simulink model "celp_ex_lsf"  (Simulink 6.1)
settings: Solver=FixedStepDiscrete  SolverMode=SingleTasking  StartTime=0.0  StopTime=300  RelTol=1e-3
PreLoadFcn:
  | load lpcvocoder.mat;
undefined symbols (not defined in the file): jet, magnitude, poly2lsf
libraries: simulink x16, dspcelplib x12, dspindex x9, dspstat3 x8, dspbuff3 x8, dspquant2 x6, dspmtrx3 x6, dsparch4 x4, dspsigops x4, dspmathops x4, dsplp x3, dspspect3 x3
(part 2 of 2)

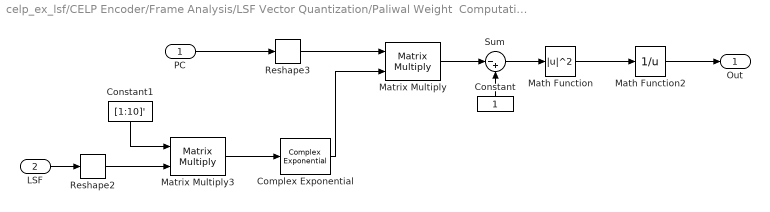
== system celp_ex_lsf/CELP Encoder/Frame Analysis/LSF Vector Quantization/Paliwal Weight  Computation/LPCpowSpec ==
  PC : Inport  Port=1  LatchInput=off
  LSF : Inport  Port=2  LatchInput=off
  Complex Exponential : dspmathops/Complex Exponential
  Constant : Constant  Orientation=up  VectorParams1D=off  SampleTime=-1
  Constant1 : Constant  Orientation=down  Value=[1:10]'  VectorParams1D=off  SampleTime=-1
  Math Function : Math  Operator=magnitude^2  SaturateOnIntegerOverflow=on
  Math Function2 : Math  Operator=reciprocal  SaturateOnIntegerOverflow=on
  Matrix Multiply : dspmtrx3/Matrix Multiply  numInputPorts=2  OptimizationLevel=None
  Matrix Multiply3 : dspmtrx3/Matrix Multiply  numInputPorts=2  OptimizationLevel=None
  Reshape2 : simulink/Math Operations/Reshape  OutputDimensionality=Row vector  OutputDimensions=[1,1]
  Reshape3 : simulink/Math Operations/Reshape  OutputDimensionality=Row vector  OutputDimensions=[1,1]
  Sum : Sum  Inputs=|-+  SaturateOnIntegerOverflow=on
  Out : Outport
  wires:
  Math Function2/1 -> Out/1
  Matrix Multiply/1 -> Sum/1
  PC/1 -> Reshape3/1
  Complex Exponential/1 -> Matrix Multiply/2
  Math Function/1 -> Math Function2/1
  Sum/1 -> Math Function/1
  Constant/1 -> Sum/2
  Reshape3/1 -> Matrix Multiply/1
  LSF/1 -> Reshape2/1
  Reshape2/1 -> Matrix Multiply3/2
  Constant1/1 -> Matrix Multiply3/1
  Matrix Multiply3/1 -> Complex Exponential/1

== system celp_ex_lsf/CELP Encoder/Subframe Analysis/Innovation signal quantization/Impulse Response/For Iterator Subsystem2 ==
  SigIn2 : Inport  Port=1  LatchInput=off
  K : Inport  Port=2  LatchInput=off
  For Iterator : ForIterator  ResetStates=reset  IterationLimit=1  ShowIterationPort=off
  Time-Varying  Synthesis Filter 1/A(z). : dsparch4/Digital Filter  DialogController=dspDDGCreate  DialogControllerArgs=DataTag6  TypePopup=IIR (all poles)  IIRFiltStruct=Direct form II transposed  AllPoleFiltStruct=Lattice AR  FIRFiltStruct=Direct form  CoeffSource=Input port(s)  NumCoeffs=[1 -.95]  DenCoeffs=[1 0.1]  BiQuadCoeffs=[1 0.3 0.4 1 0.1 0.2]  LatticeCoeffs=[0.2 0.4]  denIgnore=off  FiltPerSampPopup=One filter per frame  IC=0  ICnum=0  ICden=0  roundingMode=Floor  overflowMode=off  ScaleValues=1  scaleValueFracLength=14  stageInFracLength=15  stageOutFracLength=15
  SigOut2 : Outport
  wires:
  K/1 -> Time-Varying  Synthesis Filter 1/A(z)./2
  SigIn2/1 -> Time-Varying  Synthesis Filter 1/A(z)./1
  Time-Varying  Synthesis Filter 1/A(z)./1 -> SigOut2/1

== system celp_ex_lsf/CELP Encoder/Subframe Analysis/Innovation signal quantization/Searching for FCB pulse  positions and FCB gain/  ==
  note: This subsystem finds four FCB pulse positions and the
      | sign of the corresponding pulses based on the error between
      | the original pitch residual and its quantized version.

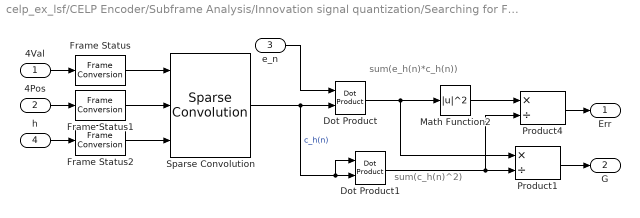
== system celp_ex_lsf/CELP Encoder/Subframe Analysis/Innovation signal quantization/Searching for FCB pulse  positions and FCB gain/Computation of  Error and Gain ==
  note: sum(e_h(n)*c_h(n))
  note: sum(c_h(n)^2)
  4Val : Inport  Port=1  LatchInput=off
  4Pos : Inport  Port=2  LatchInput=off
  e_n : Inport  Port=3  LatchInput=off
  h : Inport  Port=4  LatchInput=off
  Dot Product : simulink/Math Operations/Dot Product  OutDataType=sfix(16)  OutScaling=2^-10  DoSatur=on
  Dot Product1 : simulink/Math Operations/Dot Product  OutDataType=sfix(16)  OutScaling=2^-10  DoSatur=on
  Frame Status : FrameConversion
  Frame Status1 : FrameConversion
  Frame Status2 : FrameConversion
  Math Function2 : Math  Operator=magnitude^2  SaturateOnIntegerOverflow=on
  Product1 : Product  Inputs=*/  SaturateOnIntegerOverflow=on
  Product4 : Product  Inputs=*/  SaturateOnIntegerOverflow=on
  Sparse Convolution : dspcelplib/Sparse Convolution
  Err : Outport
  G : Outport  Port=2
  wires:
  Dot Product1/1 -> Product4/2, Product1/2
  Math Function2/1 -> Product4/1
  Dot Product/1 -> Math Function2/1, Product1/1
  Sparse Convolution/1 -> Dot Product/2, Dot Product1/2, Dot Product1/1  "c_h(n)"
  e_n/1 -> Dot Product/1
  4Val/1 -> Frame Status/1
  Product4/1 -> Err/1
  4Pos/1 -> Frame Status1/1
  h/1 -> Frame Status2/1
  Product1/1 -> G/1
  Frame Status/1 -> Sparse Convolution/1
  Frame Status1/1 -> Sparse Convolution/2
  Frame Status2/1 -> Sparse Convolution/3

== system celp_ex_lsf/CELP Encoder/Subframe Analysis/Innovation signal quantization/Searching for FCB pulse  positions and FCB gain/Optimal Features ==
  SignBit : Inport  Port=1  LatchInput=off
  Err : Inport  Port=2  LatchInput=off
  G : Inport  Port=3  LatchInput=off
  Pos : Inport  Port=4  LatchInput=off
  Data Type Conversion : DataTypeConversion  OutDataTypeMode=double  SaturateOnIntegerOverflow=on  RndMeth=Zero
  Data Type Conversion1 : DataTypeConversion  OutDataTypeMode=double  SaturateOnIntegerOverflow=on  RndMeth=Zero
  Delay1 : dspsigops/Delay  Orientation=left  dly_unit=Frames  delay=1  ic_detail=on  dif_ic_for_ch=off  dif_ic_for_dly=off  ic=0  reset_popup=None
  Feature  Concatenation : simulink/Math Operations/Matrix Concatenation  numInports=3  catMethod=Vertical
  Local maxima detector : Subsystem
  Switch : Switch  Criteria=u2 ~= 0  InputSameDT=on
  Features : Outport
  wires:
  Local maxima detector/1(Flag) -> Switch/2
  Switch/1 -> Delay1/1, Features/1
  Delay1/1 -> Switch/3
  Feature  Concatenation/1 -> Switch/1
  Data Type Conversion/1 -> Feature  Concatenation/1
  Data Type Conversion1/1 -> Feature  Concatenation/2
  Pos/1 -> Data Type Conversion/1
  SignBit/1 -> Data Type Conversion1/1
  G/1 -> Feature  Concatenation/3
  Err/1 -> Local maxima detector/1(Err)

== system celp_ex_lsf/CELP Encoder/Subframe Analysis/Innovation signal quantization/Searching for FCB pulse  positions and FCB gain/Partial decomposition of  Pitch Residual ==
  PitchRes : Inport  Port=1  LatchInput=off
  Idx : Inport  Port=2  LatchInput=off
  Control : Inport  Port=3  LatchInput=off
  Data Type Conversion : DataTypeConversion  OutDataTypeMode=double  SaturateOnIntegerOverflow=on  RndMeth=Zero
  Data Type Conversion1 : DataTypeConversion  OutDataTypeMode=int32  SaturateOnIntegerOverflow=on  RndMeth=Zero
  "Select Rows I, I+1, ...,I+3" : dspcelplib/Select Rows  numRows=4
  Sort : dspstat3/Sort  DialogController=dspDDGCreate  DialogControllerArgs=DataTag8  otype=Value  dir=Ascending  sortAlg=Quick sort  roundingMode=Floor  overflowMode=off
  Variable Selector1 : dspindex/Variable Selector  rowsOrCols=Rows  IdxMode=Variable  Elements=[1 3]  ZerOneIdxMode=One-based  errmode=Generate Error
  4Val : Outport
  4Idx : Outport  Port=2
  wires:
  Data Type Conversion1/1 -> 4Idx/1
  Idx/1 -> "Select Rows I, I+1, ...,I+3"/1
  Data Type Conversion/1 -> Sort/1
  "Select Rows I, I+1, ...,I+3"/1 -> Data Type Conversion/1
  Sort/1 -> Data Type Conversion1/1, Variable Selector1/2
  PitchRes/1 -> Variable Selector1/1
  Variable Selector1/1 -> 4Val/1
  Control/1 -> "Select Rows I, I+1, ...,I+3"/2

== system celp_ex_lsf/CELP Encoder/Subframe Analysis/Innovation signal quantization/Searching for FCB pulse  positions and FCB gain/Signal to sign bit ==
  Sig : Inport  Port=1  LatchInput=off
  Constant : Constant  Value=+1  OutDataTypeMode=int32
  Constant1 : Constant  Value=-1  OutDataTypeMode=int32
  Switch : Switch
  SignBit : Outport
  wires:
  Sig/1 -> Switch/2
  Constant1/1 -> Switch/3
  Constant/1 -> Switch/1
  Switch/1 -> SignBit/1

== system celp_ex_lsf/CELP Encoder/Subframe Analysis/Innovation signal quantization/filter/  ==
  note: This subsystem calculates the zero-state-reponse
      |
      | of the Time-Varying Synthesis Filter, 1/A(z),
      |
      | to the unquantized pitch residual signal.

== system celp_ex_lsf/CELP Encoder/Subframe Analysis/Pitch Estimation/Open loop  Pitch estimation/  ==
  note: In this subsystem, the pitch lag, D, and the optimal value of pitch gain,
      | beta, is computed. The current subframe of the residual signal is given by
      | [r(1) r(2) ... r(N)]. The mean squared error (MSE) between the current
      | subframe and the delayed-and-scaled version of this subframe (delay value,
      | D and scaling factor, beta) is given by E = sum(r(n) - beta*r(n-D)) where
      | this equation represents the summation over the whole subframe.
      |
      | The minimization of E over beta results in
      | beta = sum(r(n)*r(n-D))/ sum(r(n)*r(n)).
      |
      | The optimal beta is obtained when sum(r(n)*r(n-D))^2/ sum(r(n)*r(n))
      | is maximized.

== system celp_ex_lsf/CELP Encoder/Subframe Analysis/Pitch Estimation/Open loop  Pitch estimation/sum(r(n-D)^2) ==
  ACB : Inport  Port=1  LatchInput=off
  Autocorrelation : dspstat3/Autocorrelation  DialogController=dspDDGCreate  DialogControllerArgs=DataTag14  AllPositiveLags=off  maxlag=0  bias=None  domain=Time  roundingMode=Floor  overflowMode=off
  Constant : Constant  Orientation=up  Value=eps  VectorParams1D=off  SampleTime=-1
  For Iterator : ForIterator  IterationLimit=128
  Log all channels : dspcelplib/Log all channels  outType=Column vector  numRow=128  numCol=4  dType=double
  "Select Rows D, D+1,...D+39" : dspcelplib/Select Rows  numRows=40
  Sum3 : Sum  Inputs=|++  SaturateOnIntegerOverflow=on
  sum(r(n-D)^2) : Outport
  wires:
  Sum3/1 -> Log all channels/1
  Autocorrelation/1 -> Sum3/1
  Constant/1 -> Sum3/2
  Log all channels/1 -> sum(r(n-D)^2)/1
  [E1] -> Log all channels/2
  For Iterator/1 -> [E1], "Select Rows D, D+1,...D+39"/2  "r(n-D)"
  ACB/1 -> "Select Rows D, D+1,...D+39"/1
  "Select Rows D, D+1,...D+39"/1 -> Autocorrelation/1  "r(n-D)"

== system celp_ex_lsf/CELP Encoder/Subframe Analysis/Innovation signal quantization/Searching for FCB pulse  positions and FCB gain/Optimal Features/Local maxima detector ==
  note: Note: The 'Running Maximum' block
      | exploits the reset option in 'For' iterator
  Err : Inport  Port=1  LatchInput=off
  Relational Operator1 : RelationalOperator  Operator===  LogicOutDataTypeMode=Boolean  InputSameDT=on
  Running Maximum : dspstat3/Maximum  DialogController=dspDDGCreate  DialogControllerArgs=DataTag7  fcn=Running  reset=None  roundingMode=Floor  overflowMode=off
  Flag : Outport
  wires:
  Err/1 -> Running Maximum/1, Relational Operator1/1
  Running Maximum/1 -> Relational Operator1/2
  Relational Operator1/1 -> Flag/1
